simulink model "MainSim"  (R2024a)
settings: Solver=ode4  StartTime=0.0  StopTime=simtime  FixedStep=0.1  RelTol=1e-3
values from neighbouring files (symbols this model uses):
  C = [1 0 0 0 0 0 -1 0 0 0 0 0 ... (45 elements, 5x9)]    [C.mat]
undefined symbols (not defined in the file or in its folder): Ki, Kp, ssest, syys, utrim, xtrim
libraries: neural x680
(part 12 of 12)

== system MainSim/NARX Neural Network PSI/Layer 2/Delays 1 ==
  "p{2}" : Inport  PortDimensions=125  SampleTime=0.1
      mask Display: e = 0.06;c1 = [120 230 180]/255;c2 = ([120 230 180]+0)/(256+128);c3 = ([120 230 180]+128)/(256+128);patch([0 1 1 0],[0 0 1 1],c1);patch([0 1 1 1-e 1-e 0+e],[0 0 1 1-e 0+e 0+e],c2);patch([0 0 1 1-e 0+e 0+e],[0 1 1 1-e 1-e 0+e],c3);plot([0 1 1 0 0],[0 0 1 1 0]);
  mux : Mux  Inputs=1
      mask Display: e = 0.06;c1 = [120 150 230]/255;c2 = ([120 150 230]+0)/383;c3 = ([120 150 230]+128)/383;patch([0 1 1 0],[0 0 1 1],c1);patch([0 1 1 1-e 1-e 0+e],[0 0 1 1-e 0+e 0+e],c2);patch([0 0 1 1-e 0+e 0+e],[0 1 1 1-e 1-e 0+e],c3);plot([0 1 1 0 0],[0 0 1 1 0]);disp('Mux')
  "pd{2,1}" : Outport
      mask Display: e = 0.06;c1 = [120 230 180]/255;c2 = ([120 230 180]+0)/(256+128);c3 = ([120 230 180]+128)/(256+128);patch([0 1 1 0],[0 0 1 1],c1);patch([0 1 1 1-e 1-e 0+e],[0 0 1 1-e 0+e 0+e],c2);patch([0 0 1 1-e 0+e 0+e],[0 1 1 1-e 1-e 0+e],c3);plot([0 1 1 0 0],[0 0 1 1 0]);
  wires:
  mux/1 -> "pd{2,1}"/1
  "p{2}"/1 -> mux/1

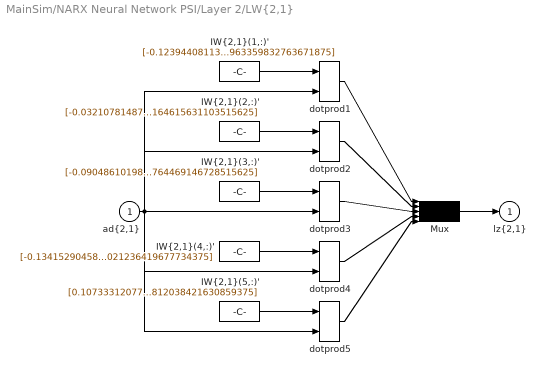
== system MainSim/NARX Neural Network PSI/Layer 2/LW{2,1} ==
  "ad{2,1}" : Inport  PortDimensions=125  SampleTime=0.1
      mask Display: e = 0.06;c1 = [120 230 180]/255;c2 = ([120 230 180]+0)/(256+128);c3 = ([120 230 180]+128)/(256+128);patch([0 1 1 0],[0 0 1 1],c1);patch([0 1 1 1-e 1-e 0+e],[0 0 1 1-e 0+e 0+e],c2);patch([0 0 1 1-e 0+e 0+e],[0 1 1 1-e 1-e 0+e],c3);plot([0 1 1 0 0],[0 0 1 1 0]);
  "IW{2,1}(1,:)'" : Constant  Value=[-0.12394408113094686207933392552149598486721515655517578125;-0.1253400431860585140242392299114726483821868896484375;0.084569388713611692853788781576440669596195220947265625;0.066178674213561772265990157393389381468296051025390625;0.1146160662897151294448150338212144561111927032470703125;0.060501719803175153800101071510653127916157245635986328125;-0.099128016447810163302989394651376642286777496337890625;0.1336829634029335356348866525877383537590503692626953125;-0.1537142888535426299423392038079327903687953948974609375;-0.054688310749235691243796964045031927525997161865234375;-0.171145329778740473702924873578012920916080474853515625;0.09382298532017628589496638369382708333432674407958984375;-0.02835004906961309523172332092144642956554889678955078125;-0.12277287236156973759815258517846814356744289398193359375;0.432454104435185338051184089636080898344516754150390625;-0.093683847480595605627939903570222668349742889404296875;0.162457470566323591842916584937484003603458404541015625;0.038936624061120951589831662431606673635542392730712890625;-0.13487275865718795220260517453425563871860504150390625;0.099761682426047659788537202985025942325592041015625;-0.1665981556666711049796703036918188445270061492919921875;0.1190298621366116249564726103926659561693668365478515625;0.0289956022517790339143584077419291133992373943328857421875;-0.12767914864125906593272929967497475445270538330078125;-0.167309546851988566462665630751871503889560699462890625;-0.2326265497019522621169329568147077225148677825927734375;-0.08068775357388442703854281035091844387352466583251953125;0.02431274780998336770831969033679342828691005706787109375;0.0519940436341362610672689470447949133813381195068359375;-0.066753715031100668841901324412901885807514190673828125;-0.01082298964401444407723573704060981981456279754638671875;-0.04803260789709910827394168109094607643783092498779296875;0.10100415529212559972993545898134470917284488677978515625;0.11503195192411093394913024212655727751553058624267578125;0.325056252053640248877997009913087822496891021728515625;0.1743849171812388576530139516762574203312397003173828125;0.2388624988318513719942615125546581111848354339599609375;-0.075830303454915870542407674292917363345623016357421875;0.1649151373221439398353282967946142889559268951416015625;-0.1076726536045460591584088660965790040791034698486328125;-0.08705907512396034164670055588430841453373432159423828125;0.10141551979669728711375142893302836455404758453369140625;0.11420109685699265933411794549101614393293857574462890625;-0.050508288100113256369194658645938034169375896453857421875;-0.1827603929120902026550510299784946255385875701904296875;0.0027420074831999929031167706483529400429688394069671630859375;0.144697445979571071017488748111645691096782684326171875;-0.06502748101242794565024496478145010769367218017578125;-0.1775412463107938487727466281285160221159458160400390625;-0.335852214481344446550536986251245252788066864013671875;0.0813243509862633662255149147313204593956470489501953125;0.114297784630717769172036923919222317636013031005859375;0.115029990623487565759575090851285494863986968994140625;-0.04521304121077047988297437086657737381756305694580078125;0.052112851456202029243325313245804863981902599334716796875;0.14653674467596478070419152572867460548877716064453125;0.458778216232629099113893289541010744869709014892578125;0.153612371769889233252825988529366441071033477783203125;0.031125169910825721542035893207867047749459743499755859375;-0.1634266258861462317586443759864778257906436920166015625;-0.043424499478260790430450555277275270782411098480224609375;0.08910620419778580991732042093644849956035614013671875;0.1559452991660345844149304639358888380229473114013671875;-0.03996341940836632689038054877528338693082332611083984375;0.0960620206044337787698594866014900617301464080810546875;0.120347959551886540818799176122411154210567474365234375;0.08977866791243678534772953980791498906910419464111328125;-0.0523049142007336598236832969632814638316631317138671875 ...(+3343 chars)]
      mask Display: e = 0.06;c1 = [120 150 230]/255;c2 = ([120 150 230]+0)/383;c3 = ([120 150 230]+128)/383;patch([0 1 1 0],[0 0 1 1],c1);patch([0 1 1 1-e 1-e 0+e],[0 0 1 1-e 0+e 0+e],c2);patch([0 0 1 1-e 0+e 0+e],[0 1 1 1-e 1-e 0+e],c3);plot([0 1 1 0 0],[0 0 1 1 0]);disp('weights');
  "IW{2,1}(2,:)'" : Constant  Value=[-0.032107814875316435798691117042835685424506664276123046875;0.0254414070444865213216356636394266388379037380218505859375;-0.09070274427646206338859968809629208408296108245849609375;0.0199906786604761473047364717103846487589180469512939453125;0.01123633229001527907009450046871279482729732990264892578125;0.08749151325219099717411808114775340072810649871826171875;-0.0957519449274308043218439934207708574831485748291015625;-0.075950106091832891852533293786109425127506256103515625;-0.10050258498128135375981884180873748846352100372314453125;0.16393815941528033786056539611308835446834564208984375;0.0735244845936481039583298979778192006051540374755859375;0.111658419175729051175949280150234699249267578125;0.11205888208569418640347947757618385367095470428466796875;0.07702151394026469921616495639682398177683353424072265625;-0.10055918933070882859137640252811252139508724212646484375;0.0449668085584356003181483174557797610759735107421875;0.04973639990417454137539010616819723509252071380615234375;0.031690744216262160815045234585340949706733226776123046875;0.0120717964269573506397303930270936689339578151702880859375;0.035145665253993409182786678002230473794043064117431640625;0.043056595037180490914696662230198853649199008941650390625;0.071525352841119771429845286547788418829441070556640625;-0.0317358134144761494521702616111724637448787689208984375;0.002448831364268749984092199412089030374772846698760986328125;-0.0150834196929737658632308949790967744775116443634033203125;-0.00576821522625250125704265968806794262491166591644287109375;0.184480194341998637863611065768054686486721038818359375;0.0175520131533726843342524404079085798002779483795166015625;0.0151502540583734190970943700449424795806407928466796875;-0.0301238050408824710457711404387737275101244449615478515625;0.0735687404186218529833496404535253532230854034423828125;-0.09655271168204453136052478612327831797301769256591796875;0.1361270693449533053520639214184484444558620452880859375;0.01184639235358669016873189860916681936942040920257568359375;0.141552252963665858853659074156894348561763763427734375;0.178277431930298491113973113897372968494892120361328125;0.071951133802321376453647872040164656937122344970703125;0.0175637720831004449928425259486175491474568843841552734375;0.05464688065709910613776401078212074935436248779296875;-0.11535871116089747856481295684716315008699893951416015625;0.0218862679976420913818824232066617696546018123626708984375;0.072789553621576297270934219341143034398555755615234375;0.10482386065656805473889079394211876206099987030029296875;0.06900053230525264591488365795157733373343944549560546875;-0.011842160340348455160874863167919102124869823455810546875;0.0917402521775950996474335852326476015150547027587890625;-0.07824748040068217613818291056304587982594966888427734375;-0.10854833332662035261240163208640296943485736846923828125;-0.09016768008047930382797829906849074177443981170654296875;-0.01647258045819162408651692430794355459511280059814453125;0.0381310627445893002285259854033938609063625335693359375;0.057118348116187704632817911942765931598842144012451171875;-0.15636242448841597418862647828063927590847015380859375;0.113157243607535595852908727465546689927577972412109375;0.0778309240262404500310111643557320348918437957763671875;0.149660633613132698638281681269290857017040252685546875;0.05759718101351507524299222495756112039089202880859375;0.08339756313810664511976256108027882874011993408203125;-0.0307558660513938819658363854614435695111751556396484375;-0.064792690401574704051057551623671315610408782958984375;0.0094058399750577802167494922969126491807401180267333984375;0.0273720034933238771934771449423351441510021686553955078125;0.08101949541561749568163719459334970451891422271728515625;-0.0715209076929385900722735414092312566936016082763671875;-0.06599595166653215994045922343502752482891082763671875;0.041311912862213522046328506576173822395503520965576171875;-0.01057099612194612077431532526361479540355503559112548828125 ...(+3407 chars)]
      mask Display: e = 0.06;c1 = [120 150 230]/255;c2 = ([120 150 230]+0)/383;c3 = ([120 150 230]+128)/383;patch([0 1 1 0],[0 0 1 1],c1);patch([0 1 1 1-e 1-e 0+e],[0 0 1 1-e 0+e 0+e],c2);patch([0 0 1 1-e 0+e 0+e],[0 1 1 1-e 1-e 0+e],c3);plot([0 1 1 0 0],[0 0 1 1 0]);disp('weights');
  "IW{2,1}(3,:)'" : Constant  Value=[-0.090486101981809563543635022142552770674228668212890625;-0.129969496361042435861321564516401849687099456787109375;0.11537473583024780710015733120599179528653621673583984375;0.1399416830397288424858714961374062113463878631591796875;0.1356760552396640562289320541822235099971294403076171875;0.1319757431654216273120283631214988417923450469970703125;-0.1056196794199042721107417719395016320049762725830078125;0.11245172656524403398403677556416369043290615081787109375;-0.09897322091315796654953373945318162441253662109375;-0.09601817827354798551287018426592112518846988677978515625;-0.142501847095443834323447163114906288683414459228515625;0.1303044883050492319664925844335812143981456756591796875;-0.1143952393049625093635057737628812901675701141357421875;-0.1103450405173499182520657768691307865083217620849609375;-0.0111753515807082835775698725910842767916619777679443359375;-0.081465272590885484671474614515318535268306732177734375;0.104425476849626941433513138690614141523838043212890625;0.1504178843301255119602188869976089335978031158447265625;-0.1052901511616907981316870746013591997325420379638671875;0.1199416552424261706022434736951254308223724365234375;-0.1167876013304449400731499508765409700572490692138671875;0.1256891917615483855730218465396319516003131866455078125;0.1479007183744875109088212639107950963079929351806640625;-0.125865757195160410386591820497415028512477874755859375;-0.09732415914220797492628634017819422297179698944091796875;-0.08876621966647879613532268194830976426601409912109375;-0.059952720677182623487677659568362287245690822601318359375;0.1576340774247453335732416235259734094142913818359375;0.11066451964965505483373675588154583238065242767333984375;-0.144856306951836211194262205026461742818355560302734375;0.1470784444346901753686296387968468479812145233154296875;-0.1435030080179618139357700101754744537174701690673828125;0.11434222276096635273479051875256118364632129669189453125;0.1348184664881851568818404984995140694081783294677734375;0.020995745354794148607169290698948316276073455810546875;0.0794164375221609597499394794795080088078975677490234375;0.1003502447073366943275374296717927791178226470947265625;-0.1427480224194247193647555604911758564412593841552734375;0.09683082316944559286842064693701104260981082916259765625;-0.10516964073577599048103792256370070390403270721435546875;-0.126788967061468416108738210823503322899341583251953125;0.1338783823361752445268990641125128604471683502197265625;0.127164896713997055410771963579463772475719451904296875;0.1606970270830817282270430723656318150460720062255859375;-0.11314299933661163544140748626887216232717037200927734375;-0.1408697174906134164107385231545777060091495513916015625;0.10353018607667506534308898835661238990724086761474609375;0.052625284372443785485540246327218483202159404754638671875;-0.0756820230522497194858289049079758115112781524658203125;-0.063755723763230187639550194944604299962520599365234375;0.13723044818511664910687386509380303323268890380859375;0.131281753537547007937291709822602570056915283203125;0.080265935563368417948737487677135504782199859619140625;-0.11266530819686837450177563368924893438816070556640625;0.14354760486774631456086126490845344960689544677734375;0.1068791826565711755581133957093697972595691680908203125;-0.0250931212901903850920337646357438643462955951690673828125;0.10864834652434741946169793891385779716074466705322265625;-0.1482855516040432475310950621860683895647525787353515625;-0.1099402743610848887101383297704160213470458984375;-0.14961939606313823247774053015746176242828369140625;0.1395605217031564981855495943818823434412479400634765625;0.11996021777157110654865590504414285533130168914794921875;-0.1479143029636794393066878683384857140481472015380859375;0.125162081736275576648864671369665302336215972900390625;0.08755269217871462783531200102515867911279201507568359375;0.1389507128122663692781912914142594672739505767822265625;0.1639080872524807108714384185077506117522716522216796875 ...(+3317 chars)]
      mask Display: e = 0.06;c1 = [120 150 230]/255;c2 = ([120 150 230]+0)/383;c3 = ([120 150 230]+128)/383;patch([0 1 1 0],[0 0 1 1],c1);patch([0 1 1 1-e 1-e 0+e],[0 0 1 1-e 0+e 0+e],c2);patch([0 0 1 1-e 0+e 0+e],[0 1 1 1-e 1-e 0+e],c3);plot([0 1 1 0 0],[0 0 1 1 0]);disp('weights');
  "IW{2,1}(4,:)'" : Constant  Value=[-0.1341529045854460699960242209272109903395175933837890625;-0.08748484792054393721638660963435540907084941864013671875;0.03660533410851864177804060318521806038916110992431640625;0.1438971984288024696940766489205998368561267852783203125;0.1298903812015861636286473412837949581444263458251953125;0.162986595185798555096567952205077745020389556884765625;-0.16721513844013380367670151827041991055011749267578125;0.035400554754196462969861869396481779403984546661376953125;-0.1569473558065044571652180138698895461857318878173828125;0.0195309222129197192219240974964122870005667209625244140625;-0.10988689725978635636227664917896618135273456573486328125;0.15833967527572934130830617505125701427459716796875;-0.020469221178140310779536292784541728906333446502685546875;-0.0166686019985660162368024117540699080564081668853759765625;-0.04463019885740109049532264862136798910796642303466796875;-0.124478458007000025720145686136675067245960235595703125;0.196404066621704120887415001561748795211315155029296875;0.1508327089905387718982154865443590097129344940185546875;-0.1108290623826846676980295569592271931469440460205078125;0.145796960146761411802884822463965974748134613037109375;-0.08832663766003480410038406489547924138605594635009765625;0.1507282972938010778829465152739430777728557586669921875;0.10924971091277267676300510856890468858182430267333984375;-0.087521504742628042361474172139423899352550506591796875;-0.1445664840160099384736014371810597367584705352783203125;-0.065451515803341020482974954575183801352977752685546875;0.02673213754010868303812031854249653406441211700439453125;0.1621628154824932277477955722133629024028778076171875;0.220781844105426561242211391800083220005035400390625;-0.1452970194165992545709542582699214108288288116455078125;0.2033694874950547626379915300276479683816432952880859375;-0.1885063858958296034717960765192401595413684844970703125;0.1758514375182454736457060562315746210515499114990234375;0.126816839937166137008972555122454650700092315673828125;0.1166503727941448909088961727320565842092037200927734375;0.1253353332062683289649385187658481299877166748046875;0.09744365766925601468617657019422040320932865142822265625;-0.11425828457004087723714036428646068088710308074951171875;0.133253757666794203640137084221350960433483123779296875;-0.170292259499640274977849685456021688878536224365234375;-0.07027966507425938147424204771596123464405536651611328125;0.1641673387859628741036743804215802811086177825927734375;0.163101778095230631748790983692742884159088134765625;0.201711541585282871924533765195519663393497467041015625;-0.12791180358132836492046635612496174871921539306640625;-0.044941083786996967319726792311485041864216327667236328125;0.0519814063660666014765610043468768708407878875732421875;0.1928451192896366850337841469809063710272312164306640625;-0.15226850468474661948192760974052362143993377685546875;-0.1138413328450109673894985462538897991180419921875;0.1507493105890818918535245529710664413869380950927734375;0.1506016576770144721475475080296746455132961273193359375;-0.03557686773899747245675229123662575148046016693115234375;-0.01420340239397631203199789950986087205819785594940185546875;0.174712804184245007466103061233297921717166900634765625;0.1483922721843186354195864851135411299765110015869140625;0.10479304877402349782666846067513688467442989349365234375;0.1578762190962714473396744097044575028121471405029296875;-0.166669968046370631231667402971652336418628692626953125;-0.1569324739784073996506919002058566547930240631103515625;-0.1279850843135716953469227519235573709011077880859375;0.1365793299096317026108948766704997979104518890380859375;0.1468789121655059981552682302208268083631992340087890625;-0.1773856393112322182847861995469429530203342437744140625;0.054619995279694834311445816865671076811850070953369140625;0.1708834916049618291022937910383916459977626800537109375;0.10919738664839140351858759458991698920726776123046875;0.2065116291186706865001809774184948764741420745849609375 ...(+3306 chars)]
      mask Display: e = 0.06;c1 = [120 150 230]/255;c2 = ([120 150 230]+0)/383;c3 = ([120 150 230]+128)/383;patch([0 1 1 0],[0 0 1 1],c1);patch([0 1 1 1-e 1-e 0+e],[0 0 1 1-e 0+e 0+e],c2);patch([0 0 1 1-e 0+e 0+e],[0 1 1 1-e 1-e 0+e],c3);plot([0 1 1 0 0],[0 0 1 1 0]);disp('weights');
  "IW{2,1}(5,:)'" : Constant  Value=[0.1073331207785641339125248805430601350963115692138671875;0.1479504677471154272527797957081929780542850494384765625;-0.19260228168033577400564126946846954524517059326171875;-0.11737315229832845364654758668621070683002471923828125;-0.12211418443315098791845940695566241629421710968017578125;-0.0920504355329767876003899118586559779942035675048828125;0.08399751868289950795798404215020127594470977783203125;-0.181683508029957696550127366208471357822418212890625;0.044418360409993522253113695796855608932673931121826171875;0.22153494484557401111857188880094327032566070556640625;0.07182425138903149319791197058293619193136692047119140625;-0.08430118210693644809072821999507141299545764923095703125;0.2179754467304171050567873635372961871325969696044921875;0.1937764343208682460417691117982030846178531646728515625;-0.096927088787803372671447732500382699072360992431640625;0.10745900872717019380875314027434797026216983795166015625;0.006293602237228450128891932280339460703544318675994873046875;-0.138874738244889550653482501729740761220455169677734375;0.121572549103653060331708957164664752781391143798828125;-0.077909183431258466345781243944657035171985626220703125;0.11697414309204288984656017191809951327741146087646484375;-0.0827128853259545826492882270031259395182132720947265625;-0.1870096860280145156796294259038404561579227447509765625;0.1435700752284465309127625687324325554072856903076171875;0.075453389121134417649727765819989144802093505859375;0.12453305408769858864115320784549112431704998016357421875;0.2038035485625623588479271575124585069715976715087890625;-0.1330138699395192192209691484094946645200252532958984375;-0.0300479265156403142766894376336495042778551578521728515625;0.1230821197090330720858020185914938338100910186767578125;-0.08074416073318223252552883195676258765161037445068359375;0.07428391886395317722513453873034450225532054901123046875;-0.024424106431571342146202852063652244396507740020751953125;-0.1248169402480973355640259114807122386991977691650390625;0.0176478346439881972340657512177131138741970062255859375;-0.03838252883591219966064045365783385932445526123046875;-0.0651695088390280563572787286830134689807891845703125;0.1598501722423608384371362944875727407634258270263671875;-0.09642879583280748734264165022977977059781551361083984375;0.04336832509398654000865036550749209709465503692626953125;0.165567281193657767079940867915865965187549591064453125;-0.07847133680189131987869899376164539717137813568115234375;-0.068109248809332445517839005333371460437774658203125;-0.1206204088588659628644705890110344626009464263916015625;0.0809605342689367624142704471523757092654705047607421875;0.2015857614742992687251188499431009404361248016357421875;-0.14771443587975863209749149973504245281219482421875;-0.047711064256893032098361118187312968075275421142578125;-0.00103490101942176385661775750435253939940594136714935302734375;0.00898758506212418532832497675144622917287051677703857421875;-0.11046361790724031071153632410641876049339771270751953125;-0.09221838461082453031192329717669053934514522552490234375;-0.2137148051007667637346543187959468923509120941162109375;0.219319020422824861871191615136922337114810943603515625;-0.0937141609096248384691563160231453366577625274658203125;-0.047093138530122612139816595799857168458402156829833984375;0.06715410840410261650301748659330769442021846771240234375;-0.057126920264274023975037408717980724759399890899658203125;0.14896644652509583028887618638691492378711700439453125;0.0558883433429337161957306534532108344137668609619140625;0.1649783140151799276651445325114764273166656494140625;-0.127067640784193525149703418719582259654998779296875;-0.0685847923415665305935107198820332996547222137451171875;0.10457966777507450573114766712023993022739887237548828125;-0.1870129979455492363893398533036815933883190155029296875;-0.04462342844665399821391105206203064881265163421630859375;-0.1551615754027177163099082690678187645971775054931640625;-0.1144728675835000319960244041794794611632823944091796875 ...(+3346 chars)]
      mask Display: e = 0.06;c1 = [120 150 230]/255;c2 = ([120 150 230]+0)/383;c3 = ([120 150 230]+128)/383;patch([0 1 1 0],[0 0 1 1],c1);patch([0 1 1 1-e 1-e 0+e],[0 0 1 1-e 0+e 0+e],c2);patch([0 0 1 1-e 0+e 0+e],[0 1 1 1-e 1-e 0+e],c3);plot([0 1 1 0 0],[0 0 1 1 0]);disp('weights');
  Mux : Mux  Inputs=5
      mask Display: e = 0.06;c1 = [120 150 230]/255;c2 = ([120 150 230]+0)/383;c3 = ([120 150 230]+128)/383;patch([0 1 1 0],[0 0 1 1],c1);patch([0 1 1 1-e 1-e 0+e],[0 0 1 1-e 0+e 0+e],c2);patch([0 0 1 1-e 0+e 0+e],[0 1 1 1-e 1-e 0+e],c3);plot([0 1 1 0 0],[0 0 1 1 0]);disp('Mux');
  dotprod{1..5} (5 alike) : neural/Weight Functions/dotprod
  "lz{2,1}" : Outport
      mask Display: e = 0.06;c1 = [120 230 180]/255;c2 = ([120 230 180]+0)/(256+128);c3 = ([120 230 180]+128)/(256+128);patch([0 1 1 0],[0 0 1 1],c1);patch([0 1 1 1-e 1-e 0+e],[0 0 1 1-e 0+e 0+e],c2);patch([0 0 1 1-e 0+e 0+e],[0 1 1 1-e 1-e 0+e],c3);plot([0 1 1 0 0],[0 0 1 1 0]);
  wires:
  Mux/1 -> "lz{2,1}"/1
  dotprod5/1 -> Mux/5
  "IW{2,1}(5,:)'"/1 -> dotprod5/1
  dotprod4/1 -> Mux/4
  "IW{2,1}(4,:)'"/1 -> dotprod4/1
  dotprod3/1 -> Mux/3
  "IW{2,1}(3,:)'"/1 -> dotprod3/1
  dotprod2/1 -> Mux/2
  "IW{2,1}(2,:)'"/1 -> dotprod2/1
  dotprod1/1 -> Mux/1
  "ad{2,1}"/1 -> dotprod5/2, dotprod4/2, dotprod3/2, dotprod2/2, dotprod1/2
  "IW{2,1}(1,:)'"/1 -> dotprod1/1

== matlab function MainSim/RCAM ==
  data: X input; XDOT output; U input
function XDOT = RCAM_model1(X,U)
% extract the state vector

x1=X(1);      % Velocity in body x axis
x2=X(2);      % Velocity in body y axis
x3=X(3);      % Velocity in body z axis
x4=X(4);      % angular rate in body x axis
x5=X(5);      % angular rate in body x axis
x6=X(6);      % angular rate in body x axis
x7=X(7);      % phi (Bank angle)
x8=X(8);      % theta (Pitch angle)
% x9=X(9);      % phi (Yaw angle)


% extract the control vector

u1=U(1);      %d_A (aileron)
u2=U(2);      %d_T (stabilizer) here the whole horizontal stabilzer moves not the elevator
u3=U(3);      %d_R (rudder)
u4=U(4);      %d_th1 (throttle 1)
u5=U(5);      %d_th2 (throttle 2)

% Nominal vehicle constants
m=120000;                   % Aircraft total mass

% NOTE:- We will define the Ib and invIb later

cbar=6.6;                  % Mean aerodynamic chord
lt=24.8;                   % Distance by AC of tail and body (m)
S=260;                     % Wing planform area (m^2)
St=64;                     % Tail planform area (m^2)

Xcg=0.23*cbar;             % X Position of cg in Fm (m)
Ycg=0;                     % Y Position of cg in Fm (m)
Zcg=0.10*cbar;             % Z Position of cg in Fm (m)

Xac=0.12*cbar;             % X position of aerodynamic center in Fm (m)
Yac=0;                     % Y position of aerodynamic center in Fm (m)
Zac=0;                     % Z position of aerodynamic center in Fm (m)

% Engine Constants
Xapt1=0;                   % X position of engine 1 force in Fm (m)
Yapt1=-7.94;               % Y position of engine 1 force in Fm (m)
Zapt1=-1.9;                % Z position of engine 1 force in Fm (m)

Xapt2=0;                   % X position of engine 2 force in Fm (m)
Yapt2=7.94;                % Y position of engine 2 force in Fm (m)
Zapt2=-1.9;                % Z position of engine 2 force in Fm (m)

% Other constants
rho             = 0.273920;          % Air density in (kg/m^3) [Cruise Altitude 38,000ft]
g               = 9.81;              % Acceleration due to gravity (m/s^2)
depsda          = 0.25;              % Change in downwash w.r.t alpha (rad/rad)
alpha_L0        = -11.5*(pi/180);    % Zero lift angle of attack (rad)
n               = 5.5;               % Slope of linear region of lift slope
a3              = -768.5;            % coefficient of alpha^3
a2              = 609.2;             % coefficient of alpha^2
a1              = -155.2;            % coefficient of alpha^1
a0              = -15.212;           % coefficient of alpha^0 (Different from RCAM Model)
alpha_switch    = 14.5*(pi/180);     % alpha value lift slope goes from linear to non-linear

% Note that these can alternatively be enforced in simulink


u1min=-15*(pi/180);
u1max=25*(pi/180);

u2min=-25*(pi/180);
u2max=10*(pi/180);

u3min=-30*(pi/180);
u3max=30*(pi/180);

u4min=0.5*(pi/180);
u4max=10*(pi/180);

u5min=0.5*(pi/180);
u5max=10*(pi/180);

if(u1>u1max)
    u1=u1max;
elseif(u1<u1min)
    u1=u1min;
end

if(u2>u2max)
    u2=u2max;
elseif(u2<u2min)
    u2=u2min;
end

if(u3>u3max)
    u3=u3max;
elseif(u3<u3min)
    u3=u3min;
end

if(u4>u4max)
    u4=u1max;
elseif(u4<u4min)
    u4=u4min;
end

if(u5>u5max)
    u5=u5max;
elseif(u5<u5min)
    u5=u5min;
end

% calculate the airspeed
Va    = sqrt(x1^2+x2^2+x3^2);

% calculate the alpha and beta
alpha = atan2(x3,x1);
beta  = asin(x2/Va);

% calculation of the dynamic pressure
Q     =0.5*rho*Va^2;

% Also define the vectors wbe_b and V_b
wbe_b = [x4;x5;x6];
V_b   = [x1;x2;x3];

% Calculate the CL_wb

if alpha<=alpha_switch

      CL_wb=n*(alpha-alpha_L0);
else
      CL_wb=a3*alpha^3+a2*alpha^2+a1*alpha+a0;
end

%Claculate CL_t

epsilon=depsda*(alpha-alpha_L0);
alpha_t=alpha-epsilon+u2+1.3*x5*lt/Va;
CL_t=3.1*(St/S)*alpha_t;

% claculation of the Total lift force
CL=CL_wb+CL_t;

% Total drag force (Neglecting the tail)
CD=0.13+0.07*(5.5*alpha+0.654)^2;

% Calculate the side force
CY=-1.6*beta+0.24*u3;

% calculate the actual dimensional forces. These are in F_s (Stability axis)

FA_s=[-CD*Q*S;CY*Q*S;-CL*Q*S];

% Rotate these forces to F_b (Body axis)
C_bs=[cos(alpha) 0 -sin(alpha);0 1 0;sin(alpha) 0 cos(alpha)];

FA_b=C_bs*FA_s;


%Calculate the moments in Fb.  Define eta,dCMdx and dCMdu

eta11=-1.4*beta;
eta21=-0.59-(3.1*(St*lt)/(S*cbar))*(alpha-epsilon);
eta31=(1-alpha*(180/(15*pi)))*beta;


eta=[eta11;eta21;eta31];

dCMdx=(cbar/Va)*[-11 0 5;0 (-4.03*(St*lt^2)/(S*cbar^2)) 0;1.7 0 -11.5]; % needed correcction

dCMdu=[-0.6 0 0.22;0 (-3.1*(St*lt)/(S*cbar)) 0;0 0 -0.63];

% Now calculate CM=[cl;cm;cn] about aerodynamic center in Fb
CMac_b=eta+dCMdx*wbe_b+dCMdu*[u1;u2;u3];

%Normalize to an aerodynamic moments

MAac_b=CMac_b*Q*S*cbar;


%Transfer moment to CG

rcg_b=[Xcg;Ycg;Zcg];
rac_b=[Xac;Yac;Zac];

MAcg_b=MAac_b+cross(FA_b,rcg_b-rac_b);

% First, calculate the thrust of each engine

F1=u4*m*g;
F2=u5*m*g;

%Assuming that the engine thrust is aligned with the Fb, we have

FE1_b=[F1;0;0];
FE2_b=[F2;0;0];

FE_b=FE1_b+FE2_b;

%Now the engine moment due to offset of engine thrust from cog

mew1=[Xcg-Xapt1;Yapt1-Ycg;Zcg-Zapt1];
mew2=[Xcg-Xapt2;Yapt2-Ycg;Zcg-Zapt2];

MEcg1_b=cross(mew1,FE1_b);
MEcg2_b=cross(mew2,FE2_b);

MEcg_b=MEcg1_b+MEcg2_b;

% Calculate the gravitational forces in the body frame. This causes no moments abot the CG


g_b=[-g*sin(x8);g*cos(x8)*sin(x7);g*cos(x8)*cos(x7)];

Fg_b=m*g_b;

%Inertia matrix

Ib=m*[40.07 0 -2.0923;0 64 0;-2.0923 0 99.92];

% Inverse of the inertia matrix

invIb=(1/m)*[0.0249836 0 0.000523151;0 0.015625 0;0.000523215 0 0.010019];


% From F_b ( all the forces in Fb ) and calculate the udot, vdot,wdot

F_b=Fg_b+FE_b+FA_b;

x1to3dot=(1/m)*F_b-cross(wbe_b,V_b);

%From Mcg_b (all the moments about the cog in Fb) and calculate pdot,qdpt,rdoot

Mcg_b=MAcg_b+MEcg_b;

x4to6dot=invIb*(Mcg_b-cross(wbe_b,Ib*wbe_b));

% Calculation of the phidot,thetadot,psidot
wbe_b1 = [x4;x5];
H_pi=[1 sin(x7)*tan(x8);0 cos(x7)];

x7to8dot=H_pi*wbe_b1;

% % Rotational Matrix from the 1 frame to 2 frame
% 
% C1v=[cos(x9) sin(x9) 0;
%     -sin(x9) cos(x9) 0;
%     0 0 1];
% 
% % Rotational Matrix from the 1 frame to 2 frame
% 
% C21=[cos(x8) 0 -sin(x8);
%     0 1 0;
%     sin(x8) 0 cos(x8)];
% 
% % Rotational Matrix from the 1 frame to 2 frame
% 
% Cb2=[1 0 0;
%     0 sin(x7) cos(x7);
%     0 -sin(x7) cos(x7)];
% 
% % Implimenting the Navigational Equation
% Cbv=Cb2*C21*C1v;
% 
% Cvb=Cbv';
% 
% x10to12dot=Cvb*V_b;

XDOT=[x1to3dot;
    x4to6dot;
    x7to8dot];
